simulink model "Calculator"  (R2024b)
settings: Solver=VariableStepAuto  StartTime=0.0  StopTime=10.0  RelTol=1e-3
(part 2 of 2)

== system Calculator/Adder7 ==
  In1 : Inport
  In2 : Inport  Port=2
  In3 : Inport  Port=3
  AND3 : Logic  IconShape=distinctive  AllPortsSameDT=off  OutDataTypeStr=boolean
  AND4 : Logic  IconShape=distinctive  AllPortsSameDT=off  OutDataTypeStr=boolean
  OR4 : Logic  Operator=OR  IconShape=distinctive  AllPortsSameDT=off  OutDataTypeStr=boolean
  XOR2 : Logic  Operator=XOR  IconShape=distinctive  AllPortsSameDT=off  OutDataTypeStr=boolean
  XOR3 : Logic  Operator=XOR  IconShape=distinctive  AllPortsSameDT=off  OutDataTypeStr=boolean
  Out1 : Outport
  Out2 : Outport  Port=2
  wires:
  In2/1 -> AND4/2, XOR2/2
  AND3/1 -> OR4/2
  In3/1 -> XOR3/2, AND3/2
  In1/1 -> AND4/1, XOR2/1
  XOR3/1 -> Out1/1
  OR4/1 -> Out2/1
  AND4/1 -> OR4/1
  XOR2/1 -> AND3/1, XOR3/1

== system Calculator/Adder8 ==
  In1 : Inport
  In2 : Inport  Port=2
  In3 : Inport  Port=3
  AND3 : Logic  IconShape=distinctive  AllPortsSameDT=off  OutDataTypeStr=boolean
  AND4 : Logic  IconShape=distinctive  AllPortsSameDT=off  OutDataTypeStr=boolean
  OR4 : Logic  Operator=OR  IconShape=distinctive  AllPortsSameDT=off  OutDataTypeStr=boolean
  XOR2 : Logic  Operator=XOR  IconShape=distinctive  AllPortsSameDT=off  OutDataTypeStr=boolean
  XOR3 : Logic  Operator=XOR  IconShape=distinctive  AllPortsSameDT=off  OutDataTypeStr=boolean
  Out : Outport
  Carry : Outport  Port=2
  wires:
  In2/1 -> AND4/2, XOR2/2
  AND3/1 -> OR4/2
  In3/1 -> XOR3/2, AND3/2
  In1/1 -> AND4/1, XOR2/1
  XOR3/1 -> Out/1
  OR4/1 -> Carry/1
  AND4/1 -> OR4/1
  XOR2/1 -> AND3/1, XOR3/1

== system Calculator/Adder9 ==
  In1 : Inport
  In2 : Inport  Port=2
  In3 : Inport  Port=3
  AND3 : Logic  IconShape=distinctive  AllPortsSameDT=off  OutDataTypeStr=boolean
  AND4 : Logic  IconShape=distinctive  AllPortsSameDT=off  OutDataTypeStr=boolean
  OR4 : Logic  Operator=OR  IconShape=distinctive  AllPortsSameDT=off  OutDataTypeStr=boolean
  XOR2 : Logic  Operator=XOR  IconShape=distinctive  AllPortsSameDT=off  OutDataTypeStr=boolean
  XOR3 : Logic  Operator=XOR  IconShape=distinctive  AllPortsSameDT=off  OutDataTypeStr=boolean
  Out : Outport
  Carry : Outport  Port=2
  wires:
  In2/1 -> AND4/2, XOR2/2
  AND3/1 -> OR4/2
  In3/1 -> XOR3/2, AND3/2
  In1/1 -> AND4/1, XOR2/1
  XOR3/1 -> Out/1
  OR4/1 -> Carry/1
  AND4/1 -> OR4/1
  XOR2/1 -> AND3/1, XOR3/1

== system Calculator/Subtractor1 ==
  In1 : Inport
  In2 : Inport  Port=2
  In3 : Inport  Port=3
  OR : Logic  Operator=OR  IconShape=distinctive  AllPortsSameDT=off  OutDataTypeStr=boolean
  Subsystem : Subsystem
  Subsystem1 : Subsystem
  Out1 : Outport
  Out2 : Outport  Port=2
  wires:
  Subsystem/1(Out1) -> Subsystem1/1(In1)
  In2/1 -> Subsystem/2(In2)
  In1/1 -> Subsystem/1(In1)
  Subsystem1/2(Out2) -> OR/1
  In3/1 -> Subsystem1/2(In2)
  Subsystem/2(Out2) -> OR/2
  Subsystem1/1(Out1) -> Out1/1
  OR/1 -> Out2/1

== system Calculator/Subtractor2 ==
  In1 : Inport
  In2 : Inport  Port=2
  In3 : Inport  Port=3
  OR : Logic  Operator=OR  IconShape=distinctive  AllPortsSameDT=off  OutDataTypeStr=boolean
  Subsystem : Subsystem
  Subsystem1 : Subsystem
  Out1 : Outport
  Out2 : Outport  Port=2
  wires:
  Subsystem/1(Out1) -> Subsystem1/1(In1)
  In2/1 -> Subsystem/2(In2)
  In1/1 -> Subsystem/1(In1)
  Subsystem1/2(Out2) -> OR/1
  In3/1 -> Subsystem1/2(In2)
  Subsystem/2(Out2) -> OR/2
  Subsystem1/1(Out1) -> Out1/1
  OR/1 -> Out2/1

== system Calculator/Subtractor3 ==
  In1 : Inport
  In2 : Inport  Port=2
  In3 : Inport  Port=3
  OR : Logic  Operator=OR  IconShape=distinctive  AllPortsSameDT=off  OutDataTypeStr=boolean
  Subsystem : Subsystem
  Subsystem1 : Subsystem
  Out1 : Outport
  Out2 : Outport  Port=2
  wires:
  Subsystem/1(Out1) -> Subsystem1/1(In1)
  In2/1 -> Subsystem/2(In2)
  In1/1 -> Subsystem/1(In1)
  Subsystem1/2(Out2) -> OR/1
  In3/1 -> Subsystem1/2(In2)
  Subsystem/2(Out2) -> OR/2
  Subsystem1/1(Out1) -> Out1/1
  OR/1 -> Out2/1

== system Calculator/Subtractor4 ==
  In1 : Inport
  In2 : Inport  Port=2
  In3 : Inport  Port=3
  OR : Logic  Operator=OR  IconShape=distinctive  AllPortsSameDT=off  OutDataTypeStr=boolean
  Subsystem : Subsystem
  Subsystem1 : Subsystem
  Out1 : Outport
  Out2 : Outport  Port=2
  wires:
  Subsystem/1(Out1) -> Subsystem1/1(In1)
  In2/1 -> Subsystem/2(In2)
  In1/1 -> Subsystem/1(In1)
  Subsystem1/2(Out2) -> OR/1
  In3/1 -> Subsystem1/2(In2)
  Subsystem/2(Out2) -> OR/2
  Subsystem1/1(Out1) -> Out1/1
  OR/1 -> Out2/1

== system Calculator/Subtractor5 ==
  In1 : Inport
  In2 : Inport  Port=2
  In3 : Inport  Port=3
  OR : Logic  Operator=OR  IconShape=distinctive  AllPortsSameDT=off  OutDataTypeStr=boolean
  Subsystem : Subsystem
  Subsystem1 : Subsystem
  Out1 : Outport
  Out2 : Outport  Port=2
  wires:
  Subsystem/1(Out1) -> Subsystem1/1(In1)
  In2/1 -> Subsystem/2(In2)
  In1/1 -> Subsystem/1(In1)
  Subsystem1/2(Out2) -> OR/1
  In3/1 -> Subsystem1/2(In2)
  Subsystem/2(Out2) -> OR/2
  Subsystem1/1(Out1) -> Out1/1
  OR/1 -> Out2/1

== system Calculator/Subtractor6 ==
  In1 : Inport
  In2 : Inport  Port=2
  In3 : Inport  Port=3
  OR : Logic  Operator=OR  IconShape=distinctive  AllPortsSameDT=off  OutDataTypeStr=boolean
  Subsystem : Subsystem
  Subsystem1 : Subsystem
  Out1 : Outport
  Out2 : Outport  Port=2
  wires:
  Subsystem/1(Out1) -> Subsystem1/1(In1)
  In2/1 -> Subsystem/2(In2)
  In1/1 -> Subsystem/1(In1)
  Subsystem1/2(Out2) -> OR/1
  In3/1 -> Subsystem1/2(In2)
  Subsystem/2(Out2) -> OR/2
  Subsystem1/1(Out1) -> Out1/1
  OR/1 -> Out2/1

== system Calculator/Subtractor7 ==
  In1 : Inport
  In2 : Inport  Port=2
  In3 : Inport  Port=3
  OR : Logic  Operator=OR  IconShape=distinctive  AllPortsSameDT=off  OutDataTypeStr=boolean
  Subsystem : Subsystem
  Subsystem1 : Subsystem
  Out1 : Outport
  Out2 : Outport  Port=2
  wires:
  Subsystem/1(Out1) -> Subsystem1/1(In1)
  In2/1 -> Subsystem/2(In2)
  In1/1 -> Subsystem/1(In1)
  Subsystem1/2(Out2) -> OR/1
  In3/1 -> Subsystem1/2(In2)
  Subsystem/2(Out2) -> OR/2
  Subsystem1/1(Out1) -> Out1/1
  OR/1 -> Out2/1

== system Calculator/Subtractor8 ==
  In1 : Inport
  In2 : Inport  Port=2
  In3 : Inport  Port=3
  OR : Logic  Operator=OR  IconShape=distinctive  AllPortsSameDT=off  OutDataTypeStr=boolean
  Subsystem : Subsystem
  Subsystem1 : Subsystem
  Out1 : Outport
  Out2 : Outport  Port=2
  wires:
  Subsystem/1(Out1) -> Subsystem1/1(In1)
  In2/1 -> Subsystem/2(In2)
  In1/1 -> Subsystem/1(In1)
  Subsystem1/2(Out2) -> OR/1
  In3/1 -> Subsystem1/2(In2)
  Subsystem/2(Out2) -> OR/2
  Subsystem1/1(Out1) -> Out1/1
  OR/1 -> Out2/1

== system Calculator/Subtractor1/Subsystem ==
  In1 : Inport
  In2 : Inport  Port=2
  AND3 : Logic  IconShape=distinctive  AllPortsSameDT=off  OutDataTypeStr=boolean
  NOT : Logic  Operator=NOT  IconShape=distinctive  AllPortsSameDT=off  OutDataTypeStr=boolean
  XOR2 : Logic  Operator=XOR  IconShape=distinctive  AllPortsSameDT=off  OutDataTypeStr=boolean
  Out1 : Outport
  Out2 : Outport  Port=2
  wires:
  In1/1 -> NOT/1, XOR2/1
  NOT/1 -> AND3/2
  AND3/1 -> Out2/1
  XOR2/1 -> Out1/1
  In2/1 -> XOR2/2, AND3/1

== system Calculator/Subtractor1/Subsystem1 ==
  In1 : Inport
  In2 : Inport  Port=2
  AND3 : Logic  IconShape=distinctive  AllPortsSameDT=off  OutDataTypeStr=boolean
  NOT : Logic  Operator=NOT  IconShape=distinctive  AllPortsSameDT=off  OutDataTypeStr=boolean
  XOR2 : Logic  Operator=XOR  IconShape=distinctive  AllPortsSameDT=off  OutDataTypeStr=boolean
  Out1 : Outport
  Out2 : Outport  Port=2
  wires:
  In1/1 -> NOT/1, XOR2/1
  NOT/1 -> AND3/2
  AND3/1 -> Out2/1
  XOR2/1 -> Out1/1
  In2/1 -> XOR2/2, AND3/1

== system Calculator/Subtractor2/Subsystem ==
  In1 : Inport
  In2 : Inport  Port=2
  AND3 : Logic  IconShape=distinctive  AllPortsSameDT=off  OutDataTypeStr=boolean
  NOT : Logic  Operator=NOT  IconShape=distinctive  AllPortsSameDT=off  OutDataTypeStr=boolean
  XOR2 : Logic  Operator=XOR  IconShape=distinctive  AllPortsSameDT=off  OutDataTypeStr=boolean
  Out1 : Outport
  Out2 : Outport  Port=2
  wires:
  In1/1 -> NOT/1, XOR2/1
  NOT/1 -> AND3/2
  AND3/1 -> Out2/1
  XOR2/1 -> Out1/1
  In2/1 -> XOR2/2, AND3/1

== system Calculator/Subtractor2/Subsystem1 ==
  In1 : Inport
  In2 : Inport  Port=2
  AND3 : Logic  IconShape=distinctive  AllPortsSameDT=off  OutDataTypeStr=boolean
  NOT : Logic  Operator=NOT  IconShape=distinctive  AllPortsSameDT=off  OutDataTypeStr=boolean
  XOR2 : Logic  Operator=XOR  IconShape=distinctive  AllPortsSameDT=off  OutDataTypeStr=boolean
  Out1 : Outport
  Out2 : Outport  Port=2
  wires:
  In1/1 -> NOT/1, XOR2/1
  NOT/1 -> AND3/2
  AND3/1 -> Out2/1
  XOR2/1 -> Out1/1
  In2/1 -> XOR2/2, AND3/1

== system Calculator/Subtractor3/Subsystem ==
  In1 : Inport
  In2 : Inport  Port=2
  AND3 : Logic  IconShape=distinctive  AllPortsSameDT=off  OutDataTypeStr=boolean
  NOT : Logic  Operator=NOT  IconShape=distinctive  AllPortsSameDT=off  OutDataTypeStr=boolean
  XOR2 : Logic  Operator=XOR  IconShape=distinctive  AllPortsSameDT=off  OutDataTypeStr=boolean
  Out1 : Outport
  Out2 : Outport  Port=2
  wires:
  In1/1 -> NOT/1, XOR2/1
  NOT/1 -> AND3/2
  AND3/1 -> Out2/1
  XOR2/1 -> Out1/1
  In2/1 -> XOR2/2, AND3/1

== system Calculator/Subtractor3/Subsystem1 ==
  In1 : Inport
  In2 : Inport  Port=2
  AND3 : Logic  IconShape=distinctive  AllPortsSameDT=off  OutDataTypeStr=boolean
  NOT : Logic  Operator=NOT  IconShape=distinctive  AllPortsSameDT=off  OutDataTypeStr=boolean
  XOR2 : Logic  Operator=XOR  IconShape=distinctive  AllPortsSameDT=off  OutDataTypeStr=boolean
  Out1 : Outport
  Out2 : Outport  Port=2
  wires:
  In1/1 -> NOT/1, XOR2/1
  NOT/1 -> AND3/2
  AND3/1 -> Out2/1
  XOR2/1 -> Out1/1
  In2/1 -> XOR2/2, AND3/1

== system Calculator/Subtractor4/Subsystem ==
  In1 : Inport
  In2 : Inport  Port=2
  AND3 : Logic  IconShape=distinctive  AllPortsSameDT=off  OutDataTypeStr=boolean
  NOT : Logic  Operator=NOT  IconShape=distinctive  AllPortsSameDT=off  OutDataTypeStr=boolean
  XOR2 : Logic  Operator=XOR  IconShape=distinctive  AllPortsSameDT=off  OutDataTypeStr=boolean
  Out1 : Outport
  Out2 : Outport  Port=2
  wires:
  In1/1 -> NOT/1, XOR2/1
  NOT/1 -> AND3/2
  AND3/1 -> Out2/1
  XOR2/1 -> Out1/1
  In2/1 -> XOR2/2, AND3/1

== system Calculator/Subtractor4/Subsystem1 ==
  In1 : Inport
  In2 : Inport  Port=2
  AND3 : Logic  IconShape=distinctive  AllPortsSameDT=off  OutDataTypeStr=boolean
  NOT : Logic  Operator=NOT  IconShape=distinctive  AllPortsSameDT=off  OutDataTypeStr=boolean
  XOR2 : Logic  Operator=XOR  IconShape=distinctive  AllPortsSameDT=off  OutDataTypeStr=boolean
  Out1 : Outport
  Out2 : Outport  Port=2
  wires:
  In1/1 -> NOT/1, XOR2/1
  NOT/1 -> AND3/2
  AND3/1 -> Out2/1
  XOR2/1 -> Out1/1
  In2/1 -> XOR2/2, AND3/1

== system Calculator/Subtractor5/Subsystem ==
  In1 : Inport
  In2 : Inport  Port=2
  AND3 : Logic  IconShape=distinctive  AllPortsSameDT=off  OutDataTypeStr=boolean
  NOT : Logic  Operator=NOT  IconShape=distinctive  AllPortsSameDT=off  OutDataTypeStr=boolean
  XOR2 : Logic  Operator=XOR  IconShape=distinctive  AllPortsSameDT=off  OutDataTypeStr=boolean
  Out1 : Outport
  Out2 : Outport  Port=2
  wires:
  In1/1 -> NOT/1, XOR2/1
  NOT/1 -> AND3/2
  AND3/1 -> Out2/1
  XOR2/1 -> Out1/1
  In2/1 -> XOR2/2, AND3/1

== system Calculator/Subtractor5/Subsystem1 ==
  In1 : Inport
  In2 : Inport  Port=2
  AND3 : Logic  IconShape=distinctive  AllPortsSameDT=off  OutDataTypeStr=boolean
  NOT : Logic  Operator=NOT  IconShape=distinctive  AllPortsSameDT=off  OutDataTypeStr=boolean
  XOR2 : Logic  Operator=XOR  IconShape=distinctive  AllPortsSameDT=off  OutDataTypeStr=boolean
  Out1 : Outport
  Out2 : Outport  Port=2
  wires:
  In1/1 -> NOT/1, XOR2/1
  NOT/1 -> AND3/2
  AND3/1 -> Out2/1
  XOR2/1 -> Out1/1
  In2/1 -> XOR2/2, AND3/1

== system Calculator/Subtractor6/Subsystem ==
  In1 : Inport
  In2 : Inport  Port=2
  AND3 : Logic  IconShape=distinctive  AllPortsSameDT=off  OutDataTypeStr=boolean
  NOT : Logic  Operator=NOT  IconShape=distinctive  AllPortsSameDT=off  OutDataTypeStr=boolean
  XOR2 : Logic  Operator=XOR  IconShape=distinctive  AllPortsSameDT=off  OutDataTypeStr=boolean
  Out1 : Outport
  Out2 : Outport  Port=2
  wires:
  In1/1 -> NOT/1, XOR2/1
  NOT/1 -> AND3/2
  AND3/1 -> Out2/1
  XOR2/1 -> Out1/1
  In2/1 -> XOR2/2, AND3/1

== system Calculator/Subtractor6/Subsystem1 ==
  In1 : Inport
  In2 : Inport  Port=2
  AND3 : Logic  IconShape=distinctive  AllPortsSameDT=off  OutDataTypeStr=boolean
  NOT : Logic  Operator=NOT  IconShape=distinctive  AllPortsSameDT=off  OutDataTypeStr=boolean
  XOR2 : Logic  Operator=XOR  IconShape=distinctive  AllPortsSameDT=off  OutDataTypeStr=boolean
  Out1 : Outport
  Out2 : Outport  Port=2
  wires:
  In1/1 -> NOT/1, XOR2/1
  NOT/1 -> AND3/2
  AND3/1 -> Out2/1
  XOR2/1 -> Out1/1
  In2/1 -> XOR2/2, AND3/1

== system Calculator/Subtractor7/Subsystem ==
  In1 : Inport
  In2 : Inport  Port=2
  AND3 : Logic  IconShape=distinctive  AllPortsSameDT=off  OutDataTypeStr=boolean
  NOT : Logic  Operator=NOT  IconShape=distinctive  AllPortsSameDT=off  OutDataTypeStr=boolean
  XOR2 : Logic  Operator=XOR  IconShape=distinctive  AllPortsSameDT=off  OutDataTypeStr=boolean
  Out1 : Outport
  Out2 : Outport  Port=2
  wires:
  In1/1 -> NOT/1, XOR2/1
  NOT/1 -> AND3/2
  AND3/1 -> Out2/1
  XOR2/1 -> Out1/1
  In2/1 -> XOR2/2, AND3/1

== system Calculator/Subtractor7/Subsystem1 ==
  In1 : Inport
  In2 : Inport  Port=2
  AND3 : Logic  IconShape=distinctive  AllPortsSameDT=off  OutDataTypeStr=boolean
  NOT : Logic  Operator=NOT  IconShape=distinctive  AllPortsSameDT=off  OutDataTypeStr=boolean
  XOR2 : Logic  Operator=XOR  IconShape=distinctive  AllPortsSameDT=off  OutDataTypeStr=boolean
  Out1 : Outport
  Out2 : Outport  Port=2
  wires:
  In1/1 -> NOT/1, XOR2/1
  NOT/1 -> AND3/2
  AND3/1 -> Out2/1
  XOR2/1 -> Out1/1
  In2/1 -> XOR2/2, AND3/1

== system Calculator/Subtractor8/Subsystem ==
  In1 : Inport
  In2 : Inport  Port=2
  AND3 : Logic  IconShape=distinctive  AllPortsSameDT=off  OutDataTypeStr=boolean
  NOT : Logic  Operator=NOT  IconShape=distinctive  AllPortsSameDT=off  OutDataTypeStr=boolean
  XOR2 : Logic  Operator=XOR  IconShape=distinctive  AllPortsSameDT=off  OutDataTypeStr=boolean
  Out1 : Outport
  Out2 : Outport  Port=2
  wires:
  In1/1 -> NOT/1, XOR2/1
  NOT/1 -> AND3/2
  AND3/1 -> Out2/1
  XOR2/1 -> Out1/1
  In2/1 -> XOR2/2, AND3/1

== system Calculator/Subtractor8/Subsystem1 ==
  In1 : Inport
  In2 : Inport  Port=2
  AND3 : Logic  IconShape=distinctive  AllPortsSameDT=off  OutDataTypeStr=boolean
  NOT : Logic  Operator=NOT  IconShape=distinctive  AllPortsSameDT=off  OutDataTypeStr=boolean
  XOR2 : Logic  Operator=XOR  IconShape=distinctive  AllPortsSameDT=off  OutDataTypeStr=boolean
  Out1 : Outport
  Out2 : Outport  Port=2
  wires:
  In1/1 -> NOT/1, XOR2/1
  NOT/1 -> AND3/2
  AND3/1 -> Out2/1
  XOR2/1 -> Out1/1
  In2/1 -> XOR2/2, AND3/1
